simulink model "anim_tp_comde_suivi_p_L"  (R2018b)
settings: Solver=ode5  StartTime=0  StopTime=36  FixedStep=.005  MaxStep=0.02  RelTol=1e-3  AbsTol=1e-6
undefined symbols (not defined in the file or in its folder): A, B, C, D, F, g, K1, L, m, M
libraries: cstblocks x1, simulink x1
Description:
  | animation stabilisation pendule inverse (modèle NL)
settings Model: Creator=user  LastModifiedBy=牟城志
settings SolverCC: AutoScaleAbsTol=off
settings DataIOCC: ExternalInput=[]  InitialState=[]  SaveFormat=Array  SignalLoggingSaveFormat=ModelDataLogs  SaveOutput=off
settings OptimizationCC: BooleanDataType=off  ExpressionDepthLimit=2147483647  InitFltsAndDblsToZero=on  LifeSpan=inf
settings DebuggingCC: SaveWithParameterizedLinksMsg=none  UnderspecifiedInitializationDetection=Classic  MergeDetectMultiDrivingBlocksExec=none  SignalResolutionControl=TryResolveAllWithWarning  MultiTaskDSMMsg=warning  MultiTaskCondExecSysMsg=none  FcnCallInpInsideContextMsg=warning  StateNameClashWarn=warning  SFUnexpectedBacktrackingDiag=warning  SFNoUnconditionalDefaultTransitionDiag=warning  SFExecutionAtInitializationDiag=none
settings HardwareCC: ProdBitPerPointer=32  ProdBitPerSizeT=32  ProdBitPerPtrDiffT=32  ProdLargestAtomicFloat=None  ProdIntDivRoundTo=Undefined  ProdEndianess=Unspecified  ProdWordSize=32  ProdHWDeviceType=32-bit Generic  TargetUnknown=on
settings ModelReferenceCC: PropagateSignalLabelsOutOfModel=off
settings SFSimCC: SimUseLocalCustomCode=off
settings RTWCC: RTWUseLocalCustomCode=off
settings CodeAppCC: StateflowObjectComments=on
settings GRTTargetCC: TargetFcnLib=ansi_tfl_tmw.mat  TargetLangStandard=C89/C90 (ANSI)  GeneratePreprocessorConditionals=Disable all  CombineOutputUpdateFcns=off  GRTInterface=on
settings ConfigComp: CovMetricSettings=dw  CovHtmlReporting=on  CovSaveCumulativeToWorkspaceVar=on  CovSaveSingleToWorkspaceVar=on  CovExternalEMLEnable=off

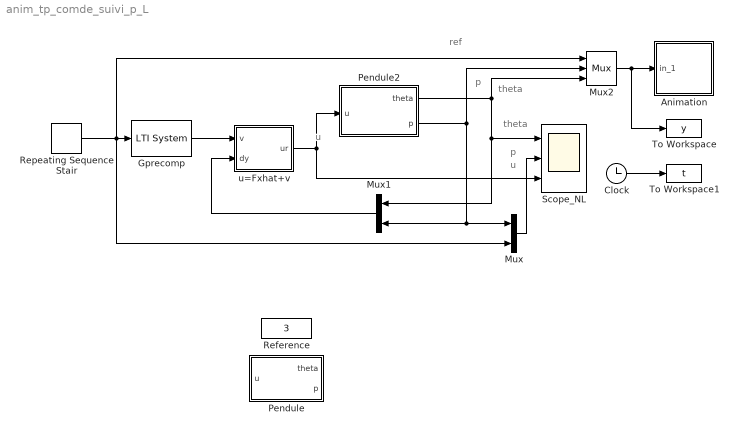
== system anim_tp_comde_suivi_p_L ==
  note: theta
  note: p
  note: theta
  note: p
  note: u
  note: u
  note: ref
  Animation : Subsystem  mask(Animation du déplacement du pendule inverse){RefBlock=Reference}
      mask prompts: RefBlock "Mask Parameter 1:"
      mask Help: Fonction d'animation du pendule inverse (voir s_fonction tp_pendan_g.m.
      mask Display: plot([-10 10],[0 0],[-2 -2 2 2],[0 1 1 0],[0 -3],[1 5])
  Clock : Clock
  Gprecomp : cstblocks/LTI System  sys=Pre  IC=[]
  Mux : Mux  Inputs=2
  Mux1 : Mux  Inputs=2
  Mux2 : Mux  Inputs=3
  Pendule : Subsystem  mask(Pendule inverse sur un chariot (éq. Linéaires).){A=A, B=B, C=C, D=D, x0=[0.1 0 0.1 0]}
      mask prompts: x0 "Conditions initiales"
      mask help: Utiliser le menu "Look under mask" pour voir les équations linéarisées de la dynamique (celles de l'énoncé du TP)
      mask Help: Description Linéarisée de la dynamique d'un pendule inverse sur un chariot.
      mask Display:
      | plot([-10 10],[1 1],[-2 -2 2 2],[1 2 2 1],[0 3],[2 5])
      | text(-12,0.5,'Eq. Linéaires')
      | plot([-14 14],[-0.5 -0.5])
  Pendule2 : Subsystem  mask(Pendule inverse sur un chariot (éq. Non Linéaires)){M=M, m=m, l=L, g=g, x0=[0.1 0 0.1 0]}
      mask prompts: M "Masse du chariot (kg):"; m "Masse du pendule (kg):"; l "Longueur de la barre (m):"; g "gravité (m/s^2):"; x0 "Conditions Initiales [theta theta' p p']"
      mask help: Utiliser le menu "Look under mask" pour voir les équations de la dynamique (celles de l'énoncé du TP)
      mask Help: Description Non Linéaire de la dynamique d'un pendule inverse sur un chariot.
      mask Display:
      | plot([-10 10],[1 1],[-2 -2 2 2],[1 2 2 1],[0 3],[2 5])
      | text(-13,0.5,'Eq. Non Linéaires')
      | plot([-14 14],[-0.5 -0.5])
  Reference : Constant  Value=3
  Repeating Sequence Stair : simulink/Sources/Repeating Sequence Stair  OutValues=[0 1 4 -2 2 0].'  tsamp=6  OutMin=[]  OutMax=[]  OutDataTypeStr=double  OutputDataTypeScalingMode=double  OutDataType=fixdt(0,8)  ConRadixGroup=Best Precision: Vector-wise  OutScaling=2^-12
  Scope_NL : Scope  NumInputPorts=3
  To Workspace : ToWorkspace  VariableName=y  SampleTime=0.1
  To Workspace1 : ToWorkspace  VariableName=t  SampleTime=0.1
  u=Fxhat+v : Subsystem
  wires:
  Mux2/1 -> To Workspace/1, Animation/1(in_1)
  Clock/1 -> To Workspace1/1
  u=Fxhat+v/1(ur) -> Pendule2/1(u), Scope_NL/3
  Mux1/1 -> u=Fxhat+v/2(dy)
  Pendule2/2(p) -> Mux/1, Mux1/2, Mux2/2
  Pendule2/1(theta) -> Scope_NL/1, Mux1/1, Mux2/3
  Gprecomp/1 -> u=Fxhat+v/1(v)
  Repeating Sequence Stair/1 -> Mux2/1, Mux/2, Gprecomp/1
  Mux/1 -> Scope_NL/2

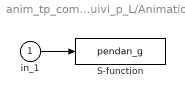
== system anim_tp_comde_suivi_p_L/Animation ==
  in_1 : Inport
  S-function : S-Function  FunctionName=pendan_g  Parameters=RefBlock  SFunctionDeploymentMode=off  EnableBusSupport=off
      settings: DeleteFcn=pendan([],[],[],'DeleteBlock');
  wires:
  in_1/1 -> S-function/1

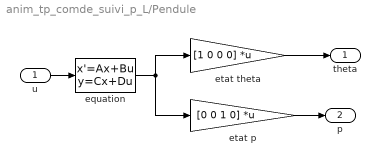
== system anim_tp_comde_suivi_p_L/Pendule ==
  u : Inport
  equation : StateSpace  A=A  B=B  C=eye(4)  D=zeros(4,1)  InitialCondition=x0
  etat p : Gain  Gain=[0 0 1 0]  Multiplication=Matrix(K*u)  SaturateOnIntegerOverflow=on  OutDataTypeStr=Inherit: Same as input  ParamDataTypeStr=Inherit: Same as input
  etat theta : Gain  Gain=[1 0 0 0]  Multiplication=Matrix(K*u)  SaturateOnIntegerOverflow=on  OutDataTypeStr=Inherit: Same as input  ParamDataTypeStr=Inherit: Same as input
  theta : Outport
  p : Outport  Port=2
  wires:
  equation/1 -> etat p/1, etat theta/1
  etat p/1 -> p/1
  u/1 -> equation/1
  etat theta/1 -> theta/1

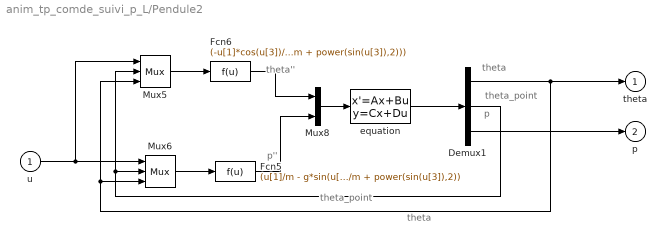
== system anim_tp_comde_suivi_p_L/Pendule2 ==
  note: p
  note: theta_point
  note: theta
  note: theta''
  note: p''
  note: theta_point
  note: theta
  u : Inport
  Demux1 : Demux  Outputs=3
  Fcn5 : Fcn  Expr=(u[1]/m - g*sin(u[3])*cos(u[3]) + l*power(u[2],2)*sin(u[3]))/(M/m + power(sin(u[3]),2))
  Fcn6 : Fcn  Expr=(-u[1]*cos(u[3])/m + (M+m)*g*sin(u[3])/m - l*power(u[2],2)*sin(u[3])*cos(u[3]))/(l*(M/m + power(sin(u[3]),2)))
  Mux5 : Mux  Inputs=3
  Mux6 : Mux  Inputs=3
  Mux8 : Mux  Inputs=2
  equation : StateSpace  A=[ 0 1 0 0 ; 0 0 0 0 ; 0 0 0 1; 0 0 0 0]  B=[0 0 ; 1 0 ; 0 0 ; 0 1]  C=[1 0 0 0 ; 0 1 0 0 ; 0 0 1 0]  D=zeros(3,2)  InitialCondition=x0
  theta : Outport  InitialOutput=0
  p : Outport  Port=2  InitialOutput=0
  wires:
  Demux1/3 -> p/1
  Demux1/1 -> theta/1, Mux5/3, Mux6/3
  Mux8/1 -> equation/1
  Fcn5/1 -> Mux8/2
  Fcn6/1 -> Mux8/1
  equation/1 -> Demux1/1
  Demux1/2 -> Mux6/2, Mux5/2
  Mux5/1 -> Fcn6/1
  Mux6/1 -> Fcn5/1
  u/1 -> Mux5/1, Mux6/1

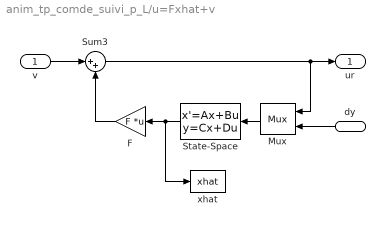
== system anim_tp_comde_suivi_p_L/u=Fxhat+v ==
  v : Inport
  dy : Inport  Port=2
  F : Gain  Gain=F  Multiplication=Matrix(K*u)  SaturateOnIntegerOverflow=on  OutDataTypeStr=Inherit: Same as input  ParamDataTypeStr=Inherit: Same as input
  Mux : Mux  Inputs=2
  State-Space : StateSpace  A=A-K1*C  B=[B K1]  C=eye(size(A,1))  D=zeros(size(A,1),size([B K1],2))  InitialCondition=0
  Sum3 : Sum  Inputs=|++  SaturateOnIntegerOverflow=on  InputSameDT=on  OutDataTypeStr=Inherit: Same as first input
  xhat : ToWorkspace  VariableName=xhat  SampleTime=-1
  ur : Outport
  wires:
  State-Space/1 -> xhat/1, F/1
  Sum3/1 -> Mux/1, ur/1
  v/1 -> Sum3/1
  Mux/1 -> State-Space/1
  dy/1 -> Mux/2
  F/1 -> Sum3/2
